simulink library "GenericINSLibrary"  (R2020b)
settings: Solver=VariableStepAuto  StartTime=0.0  StopTime=10.0  RelTol=1e-3
libraries: simulink x44
(part 4 of 6)

== system GenericINSLibrary/Sensor Fusion/SOG5 ==
  SOG : Inport
  Abs1 : Abs
  Abs2 : Abs
  Bus Selector : BusSelector  OutputSignals=measurement.timestamp
  Bus Selector1 : BusSelector  OutputSignals=measurement
  Bus Selector2 : BusSelector  OutputSignals=standardDeviation
  Bus Selector3 : BusSelector  OutputSignals=alignment
  Bus Selector4 : BusSelector  OutputSignals=positionBodyToSensor
  Bus Selector5 : BusSelector  OutputSignals=speedOverGround
  Bus Selector6 : BusSelector  OutputSignals=speedOverGround
  Data Type Conversion : DataTypeConversion  OutDataTypeStr=double
  Detect Increase : simulink/Logic and Bit Operations/Detect Increase  vinit=0.0  OutDataTypeStr=boolean
  Reshape2 : Reshape  OutputDimensionality=Customize  OutputDimensions=[3 1]
  Vector Concatenate : Concatenate
  data : Outport
  stdDev : Outport  Port=2
  sensorPosition : Outport  Port=3
  wires:
  Bus Selector6/1 -> Abs2/1  "<speedOverGround>"
  Bus Selector2/1 -> Bus Selector6/1  "<standardDeviation>"
  Bus Selector5/1 -> Abs1/1  "<speedOverGround>"
  Abs1/1 -> Vector Concatenate/2
  Reshape2/1 -> sensorPosition/1
  Abs2/1 -> stdDev/1
  Bus Selector4/1 -> Reshape2/1  "<positionBodyToSensor>"
  Bus Selector3/1 -> Bus Selector4/1  "<alignment>"
  Vector Concatenate/1 -> data/1
  Bus Selector1/1 -> Bus Selector5/1  "<measurement>"
  Detect Increase/1 -> Data Type Conversion/1
  Data Type Conversion/1 -> Vector Concatenate/1
  Bus Selector/1 -> Detect Increase/1  "<timestamp>"
  SOG/1 -> Bus Selector/1, Bus Selector1/1, Bus Selector2/1, Bus Selector3/1

== system GenericINSLibrary/Sensor Fusion/SOG6 ==
  SOG : Inport
  Abs1 : Abs
  Abs2 : Abs
  Bus Selector : BusSelector  OutputSignals=measurement.timestamp
  Bus Selector1 : BusSelector  OutputSignals=measurement
  Bus Selector2 : BusSelector  OutputSignals=standardDeviation
  Bus Selector3 : BusSelector  OutputSignals=alignment
  Bus Selector4 : BusSelector  OutputSignals=positionBodyToSensor
  Bus Selector5 : BusSelector  OutputSignals=speedOverGround
  Bus Selector6 : BusSelector  OutputSignals=speedOverGround
  Data Type Conversion : DataTypeConversion  OutDataTypeStr=double
  Detect Increase : simulink/Logic and Bit Operations/Detect Increase  vinit=0.0  OutDataTypeStr=boolean
  Reshape2 : Reshape  OutputDimensionality=Customize  OutputDimensions=[3 1]
  Vector Concatenate : Concatenate
  data : Outport
  stdDev : Outport  Port=2
  sensorPosition : Outport  Port=3
  wires:
  SOG/1 -> Bus Selector3/1, Bus Selector2/1, Bus Selector1/1, Bus Selector/1
  Bus Selector/1 -> Detect Increase/1  "<timestamp>"
  Data Type Conversion/1 -> Vector Concatenate/1
  Detect Increase/1 -> Data Type Conversion/1
  Bus Selector1/1 -> Bus Selector5/1  "<measurement>"
  Vector Concatenate/1 -> data/1
  Bus Selector3/1 -> Bus Selector4/1  "<alignment>"
  Bus Selector4/1 -> Reshape2/1  "<positionBodyToSensor>"
  Abs2/1 -> stdDev/1
  Reshape2/1 -> sensorPosition/1
  Abs1/1 -> Vector Concatenate/2
  Bus Selector5/1 -> Abs1/1  "<speedOverGround>"
  Bus Selector2/1 -> Bus Selector6/1  "<standardDeviation>"
  Bus Selector6/1 -> Abs2/1  "<speedOverGround>"

== system GenericINSLibrary/Sensor Fusion/VelocityXY1 ==
  VelocityXY : Inport
  Abs : Abs
  Bus Selector : BusSelector  OutputSignals=measurement.timestamp
  Bus Selector1 : BusSelector  OutputSignals=measurement.velocityX,measurement.velocityY  OutputAsBus=on
  Bus Selector2 : BusSelector  OutputSignals=standardDeviation  OutputAsBus=on
  Bus Selector3 : BusSelector  OutputSignals=alignment
  Bus Selector5 : BusSelector  OutputSignals=positionBodyToSensor,rotationMatrixBodyToSensor
  Bus to Vector : BusToVector
  Data Type Conversion : DataTypeConversion  OutDataTypeStr=double
  Detect Increase : simulink/Logic and Bit Operations/Detect Increase  vinit=0.0  OutDataTypeStr=boolean
  Reshape1 : Reshape  OutputDimensionality=Customize  OutputDimensions=[2 1]
  Reshape2 : Reshape  OutputDimensionality=Customize  OutputDimensions=[3 1]
  Reshape3 : Reshape  OutputDimensionality=Customize  OutputDimensions=[2 1]
  Reshape4 : Reshape  OutputDimensionality=Customize  OutputDimensions=[3 3]
  Vector Concatenate : Concatenate
  data : Outport
  stdDev : Outport  Port=2
  sensorPosition : Outport  Port=3
  sensorOrientation : Outport  Port=4
  wires:
  VelocityXY/1 -> Bus Selector3/1, Bus Selector2/1, Bus Selector1/1, Bus Selector/1
  Bus Selector/1 -> Detect Increase/1  "<timestamp>"
  Data Type Conversion/1 -> Vector Concatenate/1
  Detect Increase/1 -> Data Type Conversion/1
  Bus Selector1/1 -> Bus to Vector/1
  Bus to Vector/1 -> Reshape3/1
  Vector Concatenate/1 -> data/1
  Bus Selector2/1 -> Abs/1
  Abs/1 -> Reshape1/1
  Bus Selector3/1 -> Bus Selector5/1  "<alignment>"
  Bus Selector5/1 -> Reshape2/1  "<positionBodyToSensor>"
  Reshape3/1 -> Vector Concatenate/2
  Reshape1/1 -> stdDev/1
  Reshape2/1 -> sensorPosition/1
  Bus Selector5/2 -> Reshape4/1  "<rotationMatrixBodyToSensor>"
  Reshape4/1 -> sensorOrientation/1

== system GenericINSLibrary/Sensor Fusion/VelocityXY2 ==
  VelocityXY : Inport
  Abs : Abs
  Bus Selector : BusSelector  OutputSignals=measurement.timestamp
  Bus Selector1 : BusSelector  OutputSignals=measurement.velocityX,measurement.velocityY  OutputAsBus=on
  Bus Selector2 : BusSelector  OutputSignals=standardDeviation  OutputAsBus=on
  Bus Selector3 : BusSelector  OutputSignals=alignment
  Bus Selector5 : BusSelector  OutputSignals=positionBodyToSensor,rotationMatrixBodyToSensor
  Bus to Vector : BusToVector
  Data Type Conversion : DataTypeConversion  OutDataTypeStr=double
  Detect Increase : simulink/Logic and Bit Operations/Detect Increase  vinit=0.0  OutDataTypeStr=boolean
  Reshape1 : Reshape  OutputDimensionality=Customize  OutputDimensions=[2 1]
  Reshape2 : Reshape  OutputDimensionality=Customize  OutputDimensions=[3 1]
  Reshape3 : Reshape  OutputDimensionality=Customize  OutputDimensions=[2 1]
  Reshape4 : Reshape  OutputDimensionality=Customize  OutputDimensions=[3 3]
  Vector Concatenate : Concatenate
  data : Outport
  stdDev : Outport  Port=2
  sensorPosition : Outport  Port=3
  sensorOrientation : Outport  Port=4
  wires:
  Reshape4/1 -> sensorOrientation/1
  Bus Selector5/2 -> Reshape4/1  "<rotationMatrixBodyToSensor>"
  Reshape2/1 -> sensorPosition/1
  Reshape1/1 -> stdDev/1
  Reshape3/1 -> Vector Concatenate/2
  Bus Selector5/1 -> Reshape2/1  "<positionBodyToSensor>"
  Bus Selector3/1 -> Bus Selector5/1  "<alignment>"
  Abs/1 -> Reshape1/1
  Bus Selector2/1 -> Abs/1
  Vector Concatenate/1 -> data/1
  Bus to Vector/1 -> Reshape3/1
  Bus Selector1/1 -> Bus to Vector/1
  Detect Increase/1 -> Data Type Conversion/1
  Data Type Conversion/1 -> Vector Concatenate/1
  Bus Selector/1 -> Detect Increase/1  "<timestamp>"
  VelocityXY/1 -> Bus Selector/1, Bus Selector1/1, Bus Selector2/1, Bus Selector3/1

== system GenericINSLibrary/Sensor Fusion/VelocityXYZ1 ==
  VelocityXYZ : Inport
  Abs : Abs
  Bus Selector : BusSelector  OutputSignals=measurement.timestamp
  Bus Selector1 : BusSelector  OutputSignals=measurement.velocityX,measurement.velocityY,measurement.velocityZ  OutputAsBus=on
  Bus Selector2 : BusSelector  OutputSignals=standardDeviation  OutputAsBus=on
  Bus Selector3 : BusSelector  OutputSignals=alignment
  Bus Selector5 : BusSelector  OutputSignals=positionBodyToSensor,rotationMatrixBodyToSensor
  Bus to Vector : BusToVector
  Data Type Conversion : DataTypeConversion  OutDataTypeStr=double
  Detect Increase : simulink/Logic and Bit Operations/Detect Increase  vinit=0.0  OutDataTypeStr=boolean
  Reshape1 : Reshape  OutputDimensionality=Customize  OutputDimensions=[3 1]
  Reshape2 : Reshape  OutputDimensionality=Customize  OutputDimensions=[3 1]
  Reshape3 : Reshape  OutputDimensionality=Customize  OutputDimensions=[3 1]
  Reshape4 : Reshape  OutputDimensionality=Customize  OutputDimensions=[3 3]
  Vector Concatenate : Concatenate
  data : Outport
  stdDev : Outport  Port=2
  sensorPosition : Outport  Port=3
  sensorOrientation : Outport  Port=4
  wires:
  Reshape4/1 -> sensorOrientation/1
  Bus Selector5/2 -> Reshape4/1  "<rotationMatrixBodyToSensor>"
  Reshape2/1 -> sensorPosition/1
  Reshape1/1 -> stdDev/1
  Reshape3/1 -> Vector Concatenate/2
  Bus Selector5/1 -> Reshape2/1  "<positionBodyToSensor>"
  Bus Selector3/1 -> Bus Selector5/1  "<alignment>"
  Abs/1 -> Reshape1/1
  Bus Selector2/1 -> Abs/1
  Vector Concatenate/1 -> data/1
  Bus to Vector/1 -> Reshape3/1
  Bus Selector1/1 -> Bus to Vector/1
  Detect Increase/1 -> Data Type Conversion/1
  Data Type Conversion/1 -> Vector Concatenate/1
  Bus Selector/1 -> Detect Increase/1  "<timestamp>"
  VelocityXYZ/1 -> Bus Selector/1, Bus Selector1/1, Bus Selector2/1, Bus Selector3/1

== system GenericINSLibrary/Sensor Fusion/VelocityXYZ2 ==
  VelocityXYZ : Inport
  Abs : Abs
  Bus Selector : BusSelector  OutputSignals=measurement.timestamp
  Bus Selector1 : BusSelector  OutputSignals=measurement.velocityX,measurement.velocityY,measurement.velocityZ  OutputAsBus=on
  Bus Selector2 : BusSelector  OutputSignals=standardDeviation  OutputAsBus=on
  Bus Selector3 : BusSelector  OutputSignals=alignment
  Bus Selector5 : BusSelector  OutputSignals=positionBodyToSensor,rotationMatrixBodyToSensor
  Bus to Vector : BusToVector
  Data Type Conversion : DataTypeConversion  OutDataTypeStr=double
  Detect Increase : simulink/Logic and Bit Operations/Detect Increase  vinit=0.0  OutDataTypeStr=boolean
  Reshape1 : Reshape  OutputDimensionality=Customize  OutputDimensions=[3 1]
  Reshape2 : Reshape  OutputDimensionality=Customize  OutputDimensions=[3 1]
  Reshape3 : Reshape  OutputDimensionality=Customize  OutputDimensions=[3 1]
  Reshape4 : Reshape  OutputDimensionality=Customize  OutputDimensions=[3 3]
  Vector Concatenate : Concatenate
  data : Outport
  stdDev : Outport  Port=2
  sensorPosition : Outport  Port=3
  sensorOrientation : Outport  Port=4
  wires:
  VelocityXYZ/1 -> Bus Selector3/1, Bus Selector2/1, Bus Selector1/1, Bus Selector/1
  Bus Selector/1 -> Detect Increase/1  "<timestamp>"
  Data Type Conversion/1 -> Vector Concatenate/1
  Detect Increase/1 -> Data Type Conversion/1
  Bus Selector1/1 -> Bus to Vector/1
  Bus to Vector/1 -> Reshape3/1
  Vector Concatenate/1 -> data/1
  Bus Selector2/1 -> Abs/1
  Abs/1 -> Reshape1/1
  Bus Selector3/1 -> Bus Selector5/1  "<alignment>"
  Bus Selector5/1 -> Reshape2/1  "<positionBodyToSensor>"
  Reshape3/1 -> Vector Concatenate/2
  Reshape1/1 -> stdDev/1
  Reshape2/1 -> sensorPosition/1
  Bus Selector5/2 -> Reshape4/1  "<rotationMatrixBodyToSensor>"
  Reshape4/1 -> sensorOrientation/1

== system GenericINSLibrary/Sensor Fusion No Bias Estimation/AHRS1 ==
  AHRS : Inport
  Abs : Abs
  Bus Selector : BusSelector  OutputSignals=measurement.timestamp
  Bus Selector1 : BusSelector  OutputSignals=measurement.roll,measurement.pitch,measurement.yaw  OutputAsBus=on
  Bus Selector2 : BusSelector  OutputSignals=standardDeviation  OutputAsBus=on
  Bus Selector3 : BusSelector  OutputSignals=alignment
  Bus Selector5 : BusSelector  OutputSignals=rotationMatrixBodyToSensor
  Bus to Vector : BusToVector
  Data Type Conversion : DataTypeConversion  OutDataTypeStr=double
  Detect Increase : simulink/Logic and Bit Operations/Detect Increase  vinit=0.0  OutDataTypeStr=boolean
  Reshape1 : Reshape  OutputDimensionality=Customize  OutputDimensions=[3 1]
  Reshape3 : Reshape  OutputDimensionality=Customize  OutputDimensions=[3 1]
  Reshape4 : Reshape  OutputDimensionality=Customize  OutputDimensions=[3 3]
  Vector Concatenate : Concatenate
  data : Outport
  stdDev : Outport  Port=2
  sensorOrientation : Outport  Port=3
  wires:
  AHRS/1 -> Bus Selector3/1, Bus Selector2/1, Bus Selector1/1, Bus Selector/1
  Bus Selector/1 -> Detect Increase/1  "<timestamp>"
  Data Type Conversion/1 -> Vector Concatenate/1
  Detect Increase/1 -> Data Type Conversion/1
  Bus Selector1/1 -> Bus to Vector/1
  Bus to Vector/1 -> Reshape3/1
  Vector Concatenate/1 -> data/1
  Bus Selector2/1 -> Abs/1
  Abs/1 -> Reshape1/1
  Bus Selector3/1 -> Bus Selector5/1  "<alignment>"
  Reshape3/1 -> Vector Concatenate/2
  Reshape1/1 -> stdDev/1
  Bus Selector5/1 -> Reshape4/1  "<rotationMatrixBodyToSensor>"
  Reshape4/1 -> sensorOrientation/1

== system GenericINSLibrary/Sensor Fusion No Bias Estimation/AHRS2 ==
  AHRS : Inport
  Abs : Abs
  Bus Selector : BusSelector  OutputSignals=measurement.timestamp
  Bus Selector1 : BusSelector  OutputSignals=measurement.roll,measurement.pitch,measurement.yaw  OutputAsBus=on
  Bus Selector2 : BusSelector  OutputSignals=standardDeviation  OutputAsBus=on
  Bus Selector3 : BusSelector  OutputSignals=alignment
  Bus Selector5 : BusSelector  OutputSignals=rotationMatrixBodyToSensor
  Bus to Vector : BusToVector
  Data Type Conversion : DataTypeConversion  OutDataTypeStr=double
  Detect Increase : simulink/Logic and Bit Operations/Detect Increase  vinit=0.0  OutDataTypeStr=boolean
  Reshape1 : Reshape  OutputDimensionality=Customize  OutputDimensions=[3 1]
  Reshape3 : Reshape  OutputDimensionality=Customize  OutputDimensions=[3 1]
  Reshape4 : Reshape  OutputDimensionality=Customize  OutputDimensions=[3 3]
  Vector Concatenate : Concatenate
  data : Outport
  stdDev : Outport  Port=2
  sensorOrientation : Outport  Port=3
  wires:
  Reshape4/1 -> sensorOrientation/1
  Bus Selector5/1 -> Reshape4/1  "<rotationMatrixBodyToSensor>"
  Reshape1/1 -> stdDev/1
  Reshape3/1 -> Vector Concatenate/2
  Bus Selector3/1 -> Bus Selector5/1  "<alignment>"
  Abs/1 -> Reshape1/1
  Bus Selector2/1 -> Abs/1
  Vector Concatenate/1 -> data/1
  Bus to Vector/1 -> Reshape3/1
  Bus Selector1/1 -> Bus to Vector/1
  Detect Increase/1 -> Data Type Conversion/1
  Data Type Conversion/1 -> Vector Concatenate/1
  Bus Selector/1 -> Detect Increase/1  "<timestamp>"
  AHRS/1 -> Bus Selector/1, Bus Selector1/1, Bus Selector2/1, Bus Selector3/1

== system GenericINSLibrary/Sensor Fusion No Bias Estimation/Compass1 ==
  Compass : Inport
  Abs : Abs
  Bus Selector : BusSelector  OutputSignals=measurement.timestamp
  Bus Selector1 : BusSelector  OutputSignals=measurement.yaw
  Bus Selector2 : BusSelector  OutputSignals=standardDeviation  OutputAsBus=on
  Bus Selector3 : BusSelector  OutputSignals=alignment
  Bus Selector5 : BusSelector  OutputSignals=rotationMatrixBodyToSensor
  Data Type Conversion : DataTypeConversion  OutDataTypeStr=double
  Detect Increase : simulink/Logic and Bit Operations/Detect Increase  vinit=0.0  OutDataTypeStr=boolean
  Reshape4 : Reshape  OutputDimensionality=Customize  OutputDimensions=[3 3]
  Vector Concatenate : Concatenate
  data : Outport
  stdDev : Outport  Port=2
  sensorOrientation : Outport  Port=3
  wires:
  Reshape4/1 -> sensorOrientation/1
  Bus Selector5/1 -> Reshape4/1  "<rotationMatrixBodyToSensor>"
  Abs/1 -> stdDev/1
  Bus Selector3/1 -> Bus Selector5/1  "<alignment>"
  Bus Selector2/1 -> Abs/1
  Vector Concatenate/1 -> data/1
  Bus Selector1/1 -> Vector Concatenate/2  "<yaw>"
  Detect Increase/1 -> Data Type Conversion/1
  Data Type Conversion/1 -> Vector Concatenate/1
  Bus Selector/1 -> Detect Increase/1  "<timestamp>"
  Compass/1 -> Bus Selector/1, Bus Selector1/1, Bus Selector2/1, Bus Selector3/1

== system GenericINSLibrary/Sensor Fusion No Bias Estimation/Compass2 ==
  Compass : Inport
  Abs : Abs
  Bus Selector : BusSelector  OutputSignals=measurement.timestamp
  Bus Selector1 : BusSelector  OutputSignals=measurement.yaw
  Bus Selector2 : BusSelector  OutputSignals=standardDeviation  OutputAsBus=on
  Bus Selector3 : BusSelector  OutputSignals=alignment
  Bus Selector5 : BusSelector  OutputSignals=rotationMatrixBodyToSensor
  Data Type Conversion : DataTypeConversion  OutDataTypeStr=double
  Detect Increase : simulink/Logic and Bit Operations/Detect Increase  vinit=0.0  OutDataTypeStr=boolean
  Reshape4 : Reshape  OutputDimensionality=Customize  OutputDimensions=[3 3]
  Vector Concatenate : Concatenate
  data : Outport
  stdDev : Outport  Port=2
  sensorOrientation : Outport  Port=3
  wires:
  Compass/1 -> Bus Selector3/1, Bus Selector2/1, Bus Selector1/1, Bus Selector/1
  Bus Selector/1 -> Detect Increase/1  "<timestamp>"
  Data Type Conversion/1 -> Vector Concatenate/1
  Detect Increase/1 -> Data Type Conversion/1
  Bus Selector1/1 -> Vector Concatenate/2  "<yaw>"
  Vector Concatenate/1 -> data/1
  Bus Selector2/1 -> Abs/1
  Bus Selector3/1 -> Bus Selector5/1  "<alignment>"
  Abs/1 -> stdDev/1
  Bus Selector5/1 -> Reshape4/1  "<rotationMatrixBodyToSensor>"
  Reshape4/1 -> sensorOrientation/1

== system GenericINSLibrary/Sensor Fusion No Bias Estimation/GNSS1 ==
  GNSS : Inport
  Abs : Abs
  Bus Selector : BusSelector  OutputSignals=measurement.timestamp
  Bus Selector1 : BusSelector  OutputSignals=measurement.latitude,measurement.longitude,measurement.altitude  OutputAsBus=on
  Bus Selector2 : BusSelector  OutputSignals=standardDeviation  OutputAsBus=on
  Bus Selector3 : BusSelector  OutputSignals=alignment
  Bus Selector4 : BusSelector  OutputSignals=positionBodyToSensor
  Bus to Vector : BusToVector
  Data Type Conversion : DataTypeConversion  OutDataTypeStr=double
  Detect Increase : simulink/Logic and Bit Operations/Detect Increase  vinit=0.0  OutDataTypeStr=boolean
  Reshape1 : Reshape  OutputDimensionality=Customize  OutputDimensions=[3 1]
  Reshape2 : Reshape  OutputDimensionality=Customize  OutputDimensions=[3 1]
  Reshape3 : Reshape  OutputDimensionality=Customize  OutputDimensions=[3 1]
  Vector Concatenate : Concatenate
  data : Outport
  stdDev : Outport  Port=2
  sensorPosition : Outport  Port=3
  wires:
  GNSS/1 -> Bus Selector3/1, Bus Selector2/1, Bus Selector1/1, Bus Selector/1
  Bus Selector/1 -> Detect Increase/1  "<timestamp>"
  Data Type Conversion/1 -> Vector Concatenate/1
  Detect Increase/1 -> Data Type Conversion/1
  Bus Selector1/1 -> Bus to Vector/1
  Bus to Vector/1 -> Reshape3/1
  Vector Concatenate/1 -> data/1
  Bus Selector2/1 -> Abs/1
  Abs/1 -> Reshape1/1
  Bus Selector3/1 -> Bus Selector4/1  "<alignment>"
  Bus Selector4/1 -> Reshape2/1  "<positionBodyToSensor>"
  Reshape3/1 -> Vector Concatenate/2
  Reshape1/1 -> stdDev/1
  Reshape2/1 -> sensorPosition/1

== system GenericINSLibrary/Sensor Fusion No Bias Estimation/GNSS2 ==
  GNSS : Inport
  Abs : Abs
  Bus Selector : BusSelector  OutputSignals=measurement.timestamp
  Bus Selector1 : BusSelector  OutputSignals=measurement.latitude,measurement.longitude,measurement.altitude  OutputAsBus=on
  Bus Selector2 : BusSelector  OutputSignals=standardDeviation  OutputAsBus=on
  Bus Selector3 : BusSelector  OutputSignals=alignment
  Bus Selector4 : BusSelector  OutputSignals=positionBodyToSensor
  Bus to Vector : BusToVector
  Data Type Conversion : DataTypeConversion  OutDataTypeStr=double
  Detect Increase : simulink/Logic and Bit Operations/Detect Increase  vinit=0.0  OutDataTypeStr=boolean
  Reshape1 : Reshape  OutputDimensionality=Customize  OutputDimensions=[3 1]
  Reshape2 : Reshape  OutputDimensionality=Customize  OutputDimensions=[3 1]
  Reshape3 : Reshape  OutputDimensionality=Customize  OutputDimensions=[3 1]
  Vector Concatenate : Concatenate
  data : Outport
  stdDev : Outport  Port=2
  sensorPosition : Outport  Port=3
  wires:
  Reshape2/1 -> sensorPosition/1
  Reshape1/1 -> stdDev/1
  Reshape3/1 -> Vector Concatenate/2
  Bus Selector4/1 -> Reshape2/1  "<positionBodyToSensor>"
  Bus Selector3/1 -> Bus Selector4/1  "<alignment>"
  Abs/1 -> Reshape1/1
  Bus Selector2/1 -> Abs/1
  Vector Concatenate/1 -> data/1
  Bus to Vector/1 -> Reshape3/1
  Bus Selector1/1 -> Bus to Vector/1
  Detect Increase/1 -> Data Type Conversion/1
  Data Type Conversion/1 -> Vector Concatenate/1
  Bus Selector/1 -> Detect Increase/1  "<timestamp>"
  GNSS/1 -> Bus Selector/1, Bus Selector1/1, Bus Selector2/1, Bus Selector3/1

== system GenericINSLibrary/Sensor Fusion No Bias Estimation/GNSS3 ==
  GNSS : Inport
  Abs : Abs
  Bus Selector : BusSelector  OutputSignals=measurement.timestamp
  Bus Selector1 : BusSelector  OutputSignals=measurement.latitude,measurement.longitude,measurement.altitude  OutputAsBus=on
  Bus Selector2 : BusSelector  OutputSignals=standardDeviation  OutputAsBus=on
  Bus Selector3 : BusSelector  OutputSignals=alignment
  Bus Selector4 : BusSelector  OutputSignals=positionBodyToSensor
  Bus to Vector : BusToVector
  Data Type Conversion : DataTypeConversion  OutDataTypeStr=double
  Detect Increase : simulink/Logic and Bit Operations/Detect Increase  vinit=0.0  OutDataTypeStr=boolean
  Reshape1 : Reshape  OutputDimensionality=Customize  OutputDimensions=[3 1]
  Reshape2 : Reshape  OutputDimensionality=Customize  OutputDimensions=[3 1]
  Reshape3 : Reshape  OutputDimensionality=Customize  OutputDimensions=[3 1]
  Vector Concatenate : Concatenate
  data : Outport
  stdDev : Outport  Port=2
  sensorPosition : Outport  Port=3
  wires:
  Reshape2/1 -> sensorPosition/1
  Reshape1/1 -> stdDev/1
  Reshape3/1 -> Vector Concatenate/2
  Bus Selector4/1 -> Reshape2/1  "<positionBodyToSensor>"
  Bus Selector3/1 -> Bus Selector4/1  "<alignment>"
  Abs/1 -> Reshape1/1
  Bus Selector2/1 -> Abs/1
  Vector Concatenate/1 -> data/1
  Bus to Vector/1 -> Reshape3/1
  Bus Selector1/1 -> Bus to Vector/1
  Detect Increase/1 -> Data Type Conversion/1
  Data Type Conversion/1 -> Vector Concatenate/1
  Bus Selector/1 -> Detect Increase/1  "<timestamp>"
  GNSS/1 -> Bus Selector/1, Bus Selector1/1, Bus Selector2/1, Bus Selector3/1

== system GenericINSLibrary/Sensor Fusion No Bias Estimation/GNSS4 ==
  GNSS : Inport
  Abs : Abs
  Bus Selector : BusSelector  OutputSignals=measurement.timestamp
  Bus Selector1 : BusSelector  OutputSignals=measurement.latitude,measurement.longitude,measurement.altitude  OutputAsBus=on
  Bus Selector2 : BusSelector  OutputSignals=standardDeviation  OutputAsBus=on
  Bus Selector3 : BusSelector  OutputSignals=alignment
  Bus Selector4 : BusSelector  OutputSignals=positionBodyToSensor
  Bus to Vector : BusToVector
  Data Type Conversion : DataTypeConversion  OutDataTypeStr=double
  Detect Increase : simulink/Logic and Bit Operations/Detect Increase  vinit=0.0  OutDataTypeStr=boolean
  Reshape1 : Reshape  OutputDimensionality=Customize  OutputDimensions=[3 1]
  Reshape2 : Reshape  OutputDimensionality=Customize  OutputDimensions=[3 1]
  Reshape3 : Reshape  OutputDimensionality=Customize  OutputDimensions=[3 1]
  Vector Concatenate : Concatenate
  data : Outport
  stdDev : Outport  Port=2
  sensorPosition : Outport  Port=3
  wires:
  GNSS/1 -> Bus Selector3/1, Bus Selector2/1, Bus Selector1/1, Bus Selector/1
  Bus Selector/1 -> Detect Increase/1  "<timestamp>"
  Data Type Conversion/1 -> Vector Concatenate/1
  Detect Increase/1 -> Data Type Conversion/1
  Bus Selector1/1 -> Bus to Vector/1
  Bus to Vector/1 -> Reshape3/1
  Vector Concatenate/1 -> data/1
  Bus Selector2/1 -> Abs/1
  Abs/1 -> Reshape1/1
  Bus Selector3/1 -> Bus Selector4/1  "<alignment>"
  Bus Selector4/1 -> Reshape2/1  "<positionBodyToSensor>"
  Reshape3/1 -> Vector Concatenate/2
  Reshape1/1 -> stdDev/1
  Reshape2/1 -> sensorPosition/1

== system GenericINSLibrary/Sensor Fusion No Bias Estimation/GNSS5 ==
  GNSS : Inport
  Abs : Abs
  Bus Selector : BusSelector  OutputSignals=measurement.timestamp
  Bus Selector1 : BusSelector  OutputSignals=measurement.latitude,measurement.longitude,measurement.altitude  OutputAsBus=on
  Bus Selector2 : BusSelector  OutputSignals=standardDeviation  OutputAsBus=on
  Bus Selector3 : BusSelector  OutputSignals=alignment
  Bus Selector4 : BusSelector  OutputSignals=positionBodyToSensor
  Bus to Vector : BusToVector
  Data Type Conversion : DataTypeConversion  OutDataTypeStr=double
  Detect Increase : simulink/Logic and Bit Operations/Detect Increase  vinit=0.0  OutDataTypeStr=boolean
  Reshape1 : Reshape  OutputDimensionality=Customize  OutputDimensions=[3 1]
  Reshape2 : Reshape  OutputDimensionality=Customize  OutputDimensions=[3 1]
  Reshape3 : Reshape  OutputDimensionality=Customize  OutputDimensions=[3 1]
  Vector Concatenate : Concatenate
  data : Outport
  stdDev : Outport  Port=2
  sensorPosition : Outport  Port=3
  wires:
  GNSS/1 -> Bus Selector3/1, Bus Selector2/1, Bus Selector1/1, Bus Selector/1
  Bus Selector/1 -> Detect Increase/1  "<timestamp>"
  Data Type Conversion/1 -> Vector Concatenate/1
  Detect Increase/1 -> Data Type Conversion/1
  Bus Selector1/1 -> Bus to Vector/1
  Bus to Vector/1 -> Reshape3/1
  Vector Concatenate/1 -> data/1
  Bus Selector2/1 -> Abs/1
  Abs/1 -> Reshape1/1
  Bus Selector3/1 -> Bus Selector4/1  "<alignment>"
  Bus Selector4/1 -> Reshape2/1  "<positionBodyToSensor>"
  Reshape3/1 -> Vector Concatenate/2
  Reshape1/1 -> stdDev/1
  Reshape2/1 -> sensorPosition/1

== system GenericINSLibrary/Sensor Fusion No Bias Estimation/GNSS6 ==
  GNSS : Inport
  Abs : Abs
  Bus Selector : BusSelector  OutputSignals=measurement.timestamp
  Bus Selector1 : BusSelector  OutputSignals=measurement.latitude,measurement.longitude,measurement.altitude  OutputAsBus=on
  Bus Selector2 : BusSelector  OutputSignals=standardDeviation  OutputAsBus=on
  Bus Selector3 : BusSelector  OutputSignals=alignment
  Bus Selector4 : BusSelector  OutputSignals=positionBodyToSensor
  Bus to Vector : BusToVector
  Data Type Conversion : DataTypeConversion  OutDataTypeStr=double
  Detect Increase : simulink/Logic and Bit Operations/Detect Increase  vinit=0.0  OutDataTypeStr=boolean
  Reshape1 : Reshape  OutputDimensionality=Customize  OutputDimensions=[3 1]
  Reshape2 : Reshape  OutputDimensionality=Customize  OutputDimensions=[3 1]
  Reshape3 : Reshape  OutputDimensionality=Customize  OutputDimensions=[3 1]
  Vector Concatenate : Concatenate
  data : Outport
  stdDev : Outport  Port=2
  sensorPosition : Outport  Port=3
  wires:
  Reshape2/1 -> sensorPosition/1
  Reshape1/1 -> stdDev/1
  Reshape3/1 -> Vector Concatenate/2
  Bus Selector4/1 -> Reshape2/1  "<positionBodyToSensor>"
  Bus Selector3/1 -> Bus Selector4/1  "<alignment>"
  Abs/1 -> Reshape1/1
  Bus Selector2/1 -> Abs/1
  Vector Concatenate/1 -> data/1
  Bus to Vector/1 -> Reshape3/1
  Bus Selector1/1 -> Bus to Vector/1
  Detect Increase/1 -> Data Type Conversion/1
  Data Type Conversion/1 -> Vector Concatenate/1
  Bus Selector/1 -> Detect Increase/1  "<timestamp>"
  GNSS/1 -> Bus Selector/1, Bus Selector1/1, Bus Selector2/1, Bus Selector3/1

== system GenericINSLibrary/Sensor Fusion No Bias Estimation/IMU ==
  IMU : Inport
  Abs : Abs
  Abs1 : Abs
  Bus Selector1 : BusSelector  OutputSignals=standardDeviation  OutputAsBus=on
  Bus Selector2 : BusSelector  OutputSignals=alignment
  Bus Selector3 : BusSelector  OutputSignals=positionBodyToSensor,rotationMatrixBodyToSensor
  Bus Selector6 : BusSelector  OutputSignals=measurement.timestamp
  Bus Selector7 : BusSelector  OutputSignals=measurement.accelerationX,measurement.accelerationY,measurement.accelerationZ,measurement.angularRateX,measurement.angularRateY,measurement.angularRateZ  OutputAsBus=on
  Bus to Vector2 : BusToVector
  Data Type Conversion : DataTypeConversion  OutDataTypeStr=double
  Detect Increase : simulink/Logic and Bit Operations/Detect Increase  vinit=0.0  OutDataTypeStr=boolean
  Enabled Subsystem : Subsystem  TreatAsAtomicUnit=on
  Reshape : Reshape  OutputDimensionality=Customize  OutputDimensions=[3 1]
  Reshape1 : Reshape  OutputDimensionality=Customize  OutputDimensions=[3 3]
  Reshape2 : Reshape  OutputDimensionality=Customize  OutputDimensions=[6 1]
  Reshape3 : Reshape  OutputDimensionality=Customize  OutputDimensions=[6 1]
  Vector Concatenate : Concatenate
  sampletime : Outport
  data : Outport  Port=2
  stdDev : Outport  Port=3
  sensorPosition : Outport  Port=4
  sensorOrientation : Outport  Port=5
  wires:
  Bus Selector7/1 -> Bus to Vector2/1
  Bus Selector6/1 -> Enabled Subsystem/1(timestamp), Detect Increase/1  "<timestamp>"
  Enabled Subsystem/1(sampletime) -> Abs1/1
  IMU/1 -> Bus Selector2/1, Bus Selector1/1, Bus Selector6/1, Bus Selector7/1
  Vector Concatenate/1 -> data/1
  Bus to Vector2/1 -> Reshape3/1
  Detect Increase/1 -> Data Type Conversion/1, Enabled Subsystem/Enable
  Data Type Conversion/1 -> Vector Concatenate/1
  Bus Selector1/1 -> Abs/1
  Abs/1 -> Reshape2/1
  Bus Selector2/1 -> Bus Selector3/1  "<alignment>"
  Bus Selector3/1 -> Reshape/1  "<positionBodyToSensor>"
  Bus Selector3/2 -> Reshape1/1  "<rotationMatrixBodyToSensor>"
  Reshape/1 -> sensorPosition/1
  Reshape1/1 -> sensorOrientation/1
  Reshape2/1 -> stdDev/1
  Reshape3/1 -> Vector Concatenate/2
  Abs1/1 -> sampletime/1

== system GenericINSLibrary/Sensor Fusion No Bias Estimation/SOG1 ==
  SOG : Inport
  Abs1 : Abs
  Abs2 : Abs
  Bus Selector : BusSelector  OutputSignals=measurement.timestamp
  Bus Selector1 : BusSelector  OutputSignals=measurement
  Bus Selector2 : BusSelector  OutputSignals=standardDeviation
  Bus Selector3 : BusSelector  OutputSignals=alignment
  Bus Selector4 : BusSelector  OutputSignals=positionBodyToSensor
  Bus Selector5 : BusSelector  OutputSignals=speedOverGround
  Bus Selector6 : BusSelector  OutputSignals=speedOverGround
  Data Type Conversion : DataTypeConversion  OutDataTypeStr=double
  Detect Increase : simulink/Logic and Bit Operations/Detect Increase  vinit=0.0  OutDataTypeStr=boolean
  Reshape2 : Reshape  OutputDimensionality=Customize  OutputDimensions=[3 1]
  Vector Concatenate : Concatenate
  data : Outport
  stdDev : Outport  Port=2
  sensorPosition : Outport  Port=3
  wires:
  SOG/1 -> Bus Selector3/1, Bus Selector2/1, Bus Selector1/1, Bus Selector/1
  Bus Selector/1 -> Detect Increase/1  "<timestamp>"
  Data Type Conversion/1 -> Vector Concatenate/1
  Detect Increase/1 -> Data Type Conversion/1
  Bus Selector1/1 -> Bus Selector5/1  "<measurement>"
  Vector Concatenate/1 -> data/1
  Bus Selector3/1 -> Bus Selector4/1  "<alignment>"
  Bus Selector4/1 -> Reshape2/1  "<positionBodyToSensor>"
  Abs2/1 -> stdDev/1
  Reshape2/1 -> sensorPosition/1
  Abs1/1 -> Vector Concatenate/2
  Bus Selector5/1 -> Abs1/1  "<speedOverGround>"
  Bus Selector2/1 -> Bus Selector6/1  "<standardDeviation>"
  Bus Selector6/1 -> Abs2/1  "<speedOverGround>"

== system GenericINSLibrary/Sensor Fusion No Bias Estimation/SOG2 ==
  SOG : Inport
  Abs1 : Abs
  Abs2 : Abs
  Bus Selector : BusSelector  OutputSignals=measurement.timestamp
  Bus Selector1 : BusSelector  OutputSignals=measurement
  Bus Selector2 : BusSelector  OutputSignals=standardDeviation
  Bus Selector3 : BusSelector  OutputSignals=alignment
  Bus Selector4 : BusSelector  OutputSignals=positionBodyToSensor
  Bus Selector5 : BusSelector  OutputSignals=speedOverGround
  Bus Selector6 : BusSelector  OutputSignals=speedOverGround
  Data Type Conversion : DataTypeConversion  OutDataTypeStr=double
  Detect Increase : simulink/Logic and Bit Operations/Detect Increase  vinit=0.0  OutDataTypeStr=boolean
  Reshape2 : Reshape  OutputDimensionality=Customize  OutputDimensions=[3 1]
  Vector Concatenate : Concatenate
  data : Outport
  stdDev : Outport  Port=2
  sensorPosition : Outport  Port=3
  wires:
  Bus Selector6/1 -> Abs2/1  "<speedOverGround>"
  Bus Selector2/1 -> Bus Selector6/1  "<standardDeviation>"
  Bus Selector5/1 -> Abs1/1  "<speedOverGround>"
  Abs1/1 -> Vector Concatenate/2
  Reshape2/1 -> sensorPosition/1
  Abs2/1 -> stdDev/1
  Bus Selector4/1 -> Reshape2/1  "<positionBodyToSensor>"
  Bus Selector3/1 -> Bus Selector4/1  "<alignment>"
  Vector Concatenate/1 -> data/1
  Bus Selector1/1 -> Bus Selector5/1  "<measurement>"
  Detect Increase/1 -> Data Type Conversion/1
  Data Type Conversion/1 -> Vector Concatenate/1
  Bus Selector/1 -> Detect Increase/1  "<timestamp>"
  SOG/1 -> Bus Selector/1, Bus Selector1/1, Bus Selector2/1, Bus Selector3/1

== system GenericINSLibrary/Sensor Fusion No Bias Estimation/SOG3 ==
  SOG : Inport
  Abs1 : Abs
  Abs2 : Abs
  Bus Selector : BusSelector  OutputSignals=measurement.timestamp
  Bus Selector1 : BusSelector  OutputSignals=measurement
  Bus Selector2 : BusSelector  OutputSignals=standardDeviation
  Bus Selector3 : BusSelector  OutputSignals=alignment
  Bus Selector4 : BusSelector  OutputSignals=positionBodyToSensor
  Bus Selector5 : BusSelector  OutputSignals=speedOverGround
  Bus Selector6 : BusSelector  OutputSignals=speedOverGround
  Data Type Conversion : DataTypeConversion  OutDataTypeStr=double
  Detect Increase : simulink/Logic and Bit Operations/Detect Increase  vinit=0.0  OutDataTypeStr=boolean
  Reshape2 : Reshape  OutputDimensionality=Customize  OutputDimensions=[3 1]
  Vector Concatenate : Concatenate
  data : Outport
  stdDev : Outport  Port=2
  sensorPosition : Outport  Port=3
  wires:
  Bus Selector6/1 -> Abs2/1  "<speedOverGround>"
  Bus Selector2/1 -> Bus Selector6/1  "<standardDeviation>"
  Bus Selector5/1 -> Abs1/1  "<speedOverGround>"
  Abs1/1 -> Vector Concatenate/2
  Reshape2/1 -> sensorPosition/1
  Abs2/1 -> stdDev/1
  Bus Selector4/1 -> Reshape2/1  "<positionBodyToSensor>"
  Bus Selector3/1 -> Bus Selector4/1  "<alignment>"
  Vector Concatenate/1 -> data/1
  Bus Selector1/1 -> Bus Selector5/1  "<measurement>"
  Detect Increase/1 -> Data Type Conversion/1
  Data Type Conversion/1 -> Vector Concatenate/1
  Bus Selector/1 -> Detect Increase/1  "<timestamp>"
  SOG/1 -> Bus Selector/1, Bus Selector1/1, Bus Selector2/1, Bus Selector3/1

== system GenericINSLibrary/Sensor Fusion No Bias Estimation/SOG4 ==
  SOG : Inport
  Abs1 : Abs
  Abs2 : Abs
  Bus Selector : BusSelector  OutputSignals=measurement.timestamp
  Bus Selector1 : BusSelector  OutputSignals=measurement
  Bus Selector2 : BusSelector  OutputSignals=standardDeviation
  Bus Selector3 : BusSelector  OutputSignals=alignment
  Bus Selector4 : BusSelector  OutputSignals=positionBodyToSensor
  Bus Selector5 : BusSelector  OutputSignals=speedOverGround
  Bus Selector6 : BusSelector  OutputSignals=speedOverGround
  Data Type Conversion : DataTypeConversion  OutDataTypeStr=double
  Detect Increase : simulink/Logic and Bit Operations/Detect Increase  vinit=0.0  OutDataTypeStr=boolean
  Reshape2 : Reshape  OutputDimensionality=Customize  OutputDimensions=[3 1]
  Vector Concatenate : Concatenate
  data : Outport
  stdDev : Outport  Port=2
  sensorPosition : Outport  Port=3
  wires:
  SOG/1 -> Bus Selector3/1, Bus Selector2/1, Bus Selector1/1, Bus Selector/1
  Bus Selector/1 -> Detect Increase/1  "<timestamp>"
  Data Type Conversion/1 -> Vector Concatenate/1
  Detect Increase/1 -> Data Type Conversion/1
  Bus Selector1/1 -> Bus Selector5/1  "<measurement>"
  Vector Concatenate/1 -> data/1
  Bus Selector3/1 -> Bus Selector4/1  "<alignment>"
  Bus Selector4/1 -> Reshape2/1  "<positionBodyToSensor>"
  Abs2/1 -> stdDev/1
  Reshape2/1 -> sensorPosition/1
  Abs1/1 -> Vector Concatenate/2
  Bus Selector5/1 -> Abs1/1  "<speedOverGround>"
  Bus Selector2/1 -> Bus Selector6/1  "<standardDeviation>"
  Bus Selector6/1 -> Abs2/1  "<speedOverGround>"

== system GenericINSLibrary/Sensor Fusion No Bias Estimation/SOG5 ==
  SOG : Inport
  Abs1 : Abs
  Abs2 : Abs
  Bus Selector : BusSelector  OutputSignals=measurement.timestamp
  Bus Selector1 : BusSelector  OutputSignals=measurement
  Bus Selector2 : BusSelector  OutputSignals=standardDeviation
  Bus Selector3 : BusSelector  OutputSignals=alignment
  Bus Selector4 : BusSelector  OutputSignals=positionBodyToSensor
  Bus Selector5 : BusSelector  OutputSignals=speedOverGround
  Bus Selector6 : BusSelector  OutputSignals=speedOverGround
  Data Type Conversion : DataTypeConversion  OutDataTypeStr=double
  Detect Increase : simulink/Logic and Bit Operations/Detect Increase  vinit=0.0  OutDataTypeStr=boolean
  Reshape2 : Reshape  OutputDimensionality=Customize  OutputDimensions=[3 1]
  Vector Concatenate : Concatenate
  data : Outport
  stdDev : Outport  Port=2
  sensorPosition : Outport  Port=3
  wires:
  SOG/1 -> Bus Selector3/1, Bus Selector2/1, Bus Selector1/1, Bus Selector/1
  Bus Selector/1 -> Detect Increase/1  "<timestamp>"
  Data Type Conversion/1 -> Vector Concatenate/1
  Detect Increase/1 -> Data Type Conversion/1
  Bus Selector1/1 -> Bus Selector5/1  "<measurement>"
  Vector Concatenate/1 -> data/1
  Bus Selector3/1 -> Bus Selector4/1  "<alignment>"
  Bus Selector4/1 -> Reshape2/1  "<positionBodyToSensor>"
  Abs2/1 -> stdDev/1
  Reshape2/1 -> sensorPosition/1
  Abs1/1 -> Vector Concatenate/2
  Bus Selector5/1 -> Abs1/1  "<speedOverGround>"
  Bus Selector2/1 -> Bus Selector6/1  "<standardDeviation>"
  Bus Selector6/1 -> Abs2/1  "<speedOverGround>"

== system GenericINSLibrary/Sensor Fusion No Bias Estimation/SOG6 ==
  SOG : Inport
  Abs1 : Abs
  Abs2 : Abs
  Bus Selector : BusSelector  OutputSignals=measurement.timestamp
  Bus Selector1 : BusSelector  OutputSignals=measurement
  Bus Selector2 : BusSelector  OutputSignals=standardDeviation
  Bus Selector3 : BusSelector  OutputSignals=alignment
  Bus Selector4 : BusSelector  OutputSignals=positionBodyToSensor
  Bus Selector5 : BusSelector  OutputSignals=speedOverGround
  Bus Selector6 : BusSelector  OutputSignals=speedOverGround
  Data Type Conversion : DataTypeConversion  OutDataTypeStr=double
  Detect Increase : simulink/Logic and Bit Operations/Detect Increase  vinit=0.0  OutDataTypeStr=boolean
  Reshape2 : Reshape  OutputDimensionality=Customize  OutputDimensions=[3 1]
  Vector Concatenate : Concatenate
  data : Outport
  stdDev : Outport  Port=2
  sensorPosition : Outport  Port=3
  wires:
  Bus Selector6/1 -> Abs2/1  "<speedOverGround>"
  Bus Selector2/1 -> Bus Selector6/1  "<standardDeviation>"
  Bus Selector5/1 -> Abs1/1  "<speedOverGround>"
  Abs1/1 -> Vector Concatenate/2
  Reshape2/1 -> sensorPosition/1
  Abs2/1 -> stdDev/1
  Bus Selector4/1 -> Reshape2/1  "<positionBodyToSensor>"
  Bus Selector3/1 -> Bus Selector4/1  "<alignment>"
  Vector Concatenate/1 -> data/1
  Bus Selector1/1 -> Bus Selector5/1  "<measurement>"
  Detect Increase/1 -> Data Type Conversion/1
  Data Type Conversion/1 -> Vector Concatenate/1
  Bus Selector/1 -> Detect Increase/1  "<timestamp>"
  SOG/1 -> Bus Selector/1, Bus Selector1/1, Bus Selector2/1, Bus Selector3/1

== system GenericINSLibrary/Sensor Fusion No Bias Estimation/VelocityXY1 ==
  VelocityXY : Inport
  Abs : Abs
  Bus Selector : BusSelector  OutputSignals=measurement.timestamp
  Bus Selector1 : BusSelector  OutputSignals=measurement.velocityX,measurement.velocityY  OutputAsBus=on
  Bus Selector2 : BusSelector  OutputSignals=standardDeviation  OutputAsBus=on
  Bus Selector3 : BusSelector  OutputSignals=alignment
  Bus Selector5 : BusSelector  OutputSignals=positionBodyToSensor,rotationMatrixBodyToSensor
  Bus to Vector : BusToVector
  Data Type Conversion : DataTypeConversion  OutDataTypeStr=double
  Detect Increase : simulink/Logic and Bit Operations/Detect Increase  vinit=0.0  OutDataTypeStr=boolean
  Reshape1 : Reshape  OutputDimensionality=Customize  OutputDimensions=[2 1]
  Reshape2 : Reshape  OutputDimensionality=Customize  OutputDimensions=[3 1]
  Reshape3 : Reshape  OutputDimensionality=Customize  OutputDimensions=[2 1]
  Reshape4 : Reshape  OutputDimensionality=Customize  OutputDimensions=[3 3]
  Vector Concatenate : Concatenate
  data : Outport
  stdDev : Outport  Port=2
  sensorPosition : Outport  Port=3
  sensorOrientation : Outport  Port=4
  wires:
  Reshape4/1 -> sensorOrientation/1
  Bus Selector5/2 -> Reshape4/1  "<rotationMatrixBodyToSensor>"
  Reshape2/1 -> sensorPosition/1
  Reshape1/1 -> stdDev/1
  Reshape3/1 -> Vector Concatenate/2
  Bus Selector5/1 -> Reshape2/1  "<positionBodyToSensor>"
  Bus Selector3/1 -> Bus Selector5/1  "<alignment>"
  Abs/1 -> Reshape1/1
  Bus Selector2/1 -> Abs/1
  Vector Concatenate/1 -> data/1
  Bus to Vector/1 -> Reshape3/1
  Bus Selector1/1 -> Bus to Vector/1
  Detect Increase/1 -> Data Type Conversion/1
  Data Type Conversion/1 -> Vector Concatenate/1
  Bus Selector/1 -> Detect Increase/1  "<timestamp>"
  VelocityXY/1 -> Bus Selector/1, Bus Selector1/1, Bus Selector2/1, Bus Selector3/1

== system GenericINSLibrary/Sensor Fusion No Bias Estimation/VelocityXY2 ==
  VelocityXY : Inport
  Abs : Abs
  Bus Selector : BusSelector  OutputSignals=measurement.timestamp
  Bus Selector1 : BusSelector  OutputSignals=measurement.velocityX,measurement.velocityY  OutputAsBus=on
  Bus Selector2 : BusSelector  OutputSignals=standardDeviation  OutputAsBus=on
  Bus Selector3 : BusSelector  OutputSignals=alignment
  Bus Selector5 : BusSelector  OutputSignals=positionBodyToSensor,rotationMatrixBodyToSensor
  Bus to Vector : BusToVector
  Data Type Conversion : DataTypeConversion  OutDataTypeStr=double
  Detect Increase : simulink/Logic and Bit Operations/Detect Increase  vinit=0.0  OutDataTypeStr=boolean
  Reshape1 : Reshape  OutputDimensionality=Customize  OutputDimensions=[2 1]
  Reshape2 : Reshape  OutputDimensionality=Customize  OutputDimensions=[3 1]
  Reshape3 : Reshape  OutputDimensionality=Customize  OutputDimensions=[2 1]
  Reshape4 : Reshape  OutputDimensionality=Customize  OutputDimensions=[3 3]
  Vector Concatenate : Concatenate
  data : Outport
  stdDev : Outport  Port=2
  sensorPosition : Outport  Port=3
  sensorOrientation : Outport  Port=4
  wires:
  VelocityXY/1 -> Bus Selector3/1, Bus Selector2/1, Bus Selector1/1, Bus Selector/1
  Bus Selector/1 -> Detect Increase/1  "<timestamp>"
  Data Type Conversion/1 -> Vector Concatenate/1
  Detect Increase/1 -> Data Type Conversion/1
  Bus Selector1/1 -> Bus to Vector/1
  Bus to Vector/1 -> Reshape3/1
  Vector Concatenate/1 -> data/1
  Bus Selector2/1 -> Abs/1
  Abs/1 -> Reshape1/1
  Bus Selector3/1 -> Bus Selector5/1  "<alignment>"
  Bus Selector5/1 -> Reshape2/1  "<positionBodyToSensor>"
  Reshape3/1 -> Vector Concatenate/2
  Reshape1/1 -> stdDev/1
  Reshape2/1 -> sensorPosition/1
  Bus Selector5/2 -> Reshape4/1  "<rotationMatrixBodyToSensor>"
  Reshape4/1 -> sensorOrientation/1

== system GenericINSLibrary/Sensor Fusion No Bias Estimation/VelocityXYZ1 ==
  VelocityXYZ : Inport
  Abs : Abs
  Bus Selector : BusSelector  OutputSignals=measurement.timestamp
  Bus Selector1 : BusSelector  OutputSignals=measurement.velocityX,measurement.velocityY,measurement.velocityZ  OutputAsBus=on
  Bus Selector2 : BusSelector  OutputSignals=standardDeviation  OutputAsBus=on
  Bus Selector3 : BusSelector  OutputSignals=alignment
  Bus Selector5 : BusSelector  OutputSignals=positionBodyToSensor,rotationMatrixBodyToSensor
  Bus to Vector : BusToVector
  Data Type Conversion : DataTypeConversion  OutDataTypeStr=double
  Detect Increase : simulink/Logic and Bit Operations/Detect Increase  vinit=0.0  OutDataTypeStr=boolean
  Reshape1 : Reshape  OutputDimensionality=Customize  OutputDimensions=[3 1]
  Reshape2 : Reshape  OutputDimensionality=Customize  OutputDimensions=[3 1]
  Reshape3 : Reshape  OutputDimensionality=Customize  OutputDimensions=[3 1]
  Reshape4 : Reshape  OutputDimensionality=Customize  OutputDimensions=[3 3]
  Vector Concatenate : Concatenate
  data : Outport
  stdDev : Outport  Port=2
  sensorPosition : Outport  Port=3
  sensorOrientation : Outport  Port=4
  wires:
  VelocityXYZ/1 -> Bus Selector3/1, Bus Selector2/1, Bus Selector1/1, Bus Selector/1
  Bus Selector/1 -> Detect Increase/1  "<timestamp>"
  Data Type Conversion/1 -> Vector Concatenate/1
  Detect Increase/1 -> Data Type Conversion/1
  Bus Selector1/1 -> Bus to Vector/1
  Bus to Vector/1 -> Reshape3/1
  Vector Concatenate/1 -> data/1
  Bus Selector2/1 -> Abs/1
  Abs/1 -> Reshape1/1
  Bus Selector3/1 -> Bus Selector5/1  "<alignment>"
  Bus Selector5/1 -> Reshape2/1  "<positionBodyToSensor>"
  Reshape3/1 -> Vector Concatenate/2
  Reshape1/1 -> stdDev/1
  Reshape2/1 -> sensorPosition/1
  Bus Selector5/2 -> Reshape4/1  "<rotationMatrixBodyToSensor>"
  Reshape4/1 -> sensorOrientation/1

== system GenericINSLibrary/Sensor Fusion No Bias Estimation/VelocityXYZ2 ==
  VelocityXYZ : Inport
  Abs : Abs
  Bus Selector : BusSelector  OutputSignals=measurement.timestamp
  Bus Selector1 : BusSelector  OutputSignals=measurement.velocityX,measurement.velocityY,measurement.velocityZ  OutputAsBus=on
  Bus Selector2 : BusSelector  OutputSignals=standardDeviation  OutputAsBus=on
  Bus Selector3 : BusSelector  OutputSignals=alignment
  Bus Selector5 : BusSelector  OutputSignals=positionBodyToSensor,rotationMatrixBodyToSensor
  Bus to Vector : BusToVector
  Data Type Conversion : DataTypeConversion  OutDataTypeStr=double
  Detect Increase : simulink/Logic and Bit Operations/Detect Increase  vinit=0.0  OutDataTypeStr=boolean
  Reshape1 : Reshape  OutputDimensionality=Customize  OutputDimensions=[3 1]
  Reshape2 : Reshape  OutputDimensionality=Customize  OutputDimensions=[3 1]
  Reshape3 : Reshape  OutputDimensionality=Customize  OutputDimensions=[3 1]
  Reshape4 : Reshape  OutputDimensionality=Customize  OutputDimensions=[3 3]
  Vector Concatenate : Concatenate
  data : Outport
  stdDev : Outport  Port=2
  sensorPosition : Outport  Port=3
  sensorOrientation : Outport  Port=4
  wires:
  Reshape4/1 -> sensorOrientation/1
  Bus Selector5/2 -> Reshape4/1  "<rotationMatrixBodyToSensor>"
  Reshape2/1 -> sensorPosition/1
  Reshape1/1 -> stdDev/1
  Reshape3/1 -> Vector Concatenate/2
  Bus Selector5/1 -> Reshape2/1  "<positionBodyToSensor>"
  Bus Selector3/1 -> Bus Selector5/1  "<alignment>"
  Abs/1 -> Reshape1/1
  Bus Selector2/1 -> Abs/1
  Vector Concatenate/1 -> data/1
  Bus to Vector/1 -> Reshape3/1
  Bus Selector1/1 -> Bus to Vector/1
  Detect Increase/1 -> Data Type Conversion/1
  Data Type Conversion/1 -> Vector Concatenate/1
  Bus Selector/1 -> Detect Increase/1  "<timestamp>"
  VelocityXYZ/1 -> Bus Selector/1, Bus Selector1/1, Bus Selector2/1, Bus Selector3/1

== system GenericINSLibrary/Sensor Fusion/IMU/Enabled Subsystem ==
  timestamp : Inport
  Enable : EnablePort
  Difference : simulink/Discrete/Difference  ICPrevInput=0.0  OutMin=[]  OutMax=[]  OutDataType=fixdt(1, 16)  OutScaling=2^-10  DoSatur=off
  sampletime : Outport
  wires:
  Difference/1 -> sampletime/1
  timestamp/1 -> Difference/1

== system GenericINSLibrary/Sensor Fusion No Bias Estimation/IMU/Enabled Subsystem ==
  timestamp : Inport
  Enable : EnablePort
  Difference : simulink/Discrete/Difference  ICPrevInput=0.0  OutMin=[]  OutMax=[]  OutDataType=fixdt(1, 16)  OutScaling=2^-10  DoSatur=off
  sampletime : Outport
  wires:
  timestamp/1 -> Difference/1
  Difference/1 -> sampletime/1
